simulink model "StateSpaceExe"  (R2018b)
settings: Solver=VariableStepAuto  StartTime=0.0  StopTime=100  RelTol=1e-3
values from neighbouring files (symbols this model uses):
  A = [-7.6258  0; 1  0]    [stateSpace.mat]    (also in stateSpaceData.mat; stateSpaceDataAntiWindup.mat)
  B = [1 0]    [stateSpace.mat]    (also in stateSpaceData.mat; stateSpaceDataAntiWindup.mat)
  C = [0 162.7435]    [stateSpace.mat]    (also in stateSpaceData.mat; stateSpaceDataAntiWindup.mat)
  D = 0    [stateSpace.mat]    (also in stateSpaceData.mat; stateSpaceDataAntiWindup.mat)
  K = [-3.4258 5.6 -0.014747132758]    [stateSpace.mat]    (also in stateSpaceData.mat = [-3.4258 5.6]; stateSpaceDataAntiWindup.mat = [82.3742 2600]; toStateSpace.m = [Kx(1) Kx(2)])
  Ki = -0.014747132758    [stateSpaceData.mat]    (also in stateSpaceDataAntiWindup.mat = 147.47132758; toStateSpace.m = Kx(3))
  L = [3.35099850771 0.334109810837]    [stateSpace.mat]    (also in stateSpaceData.mat = [0.0638134588478 0.0883242648708]; stateSpaceDataAntiWindup.mat = [191.93766157 2.22665851478]; toStateSpace.m = acker(A', C', [polo1, polo2])')
settings Model: Creator=lucas  LastModifiedBy=lucas

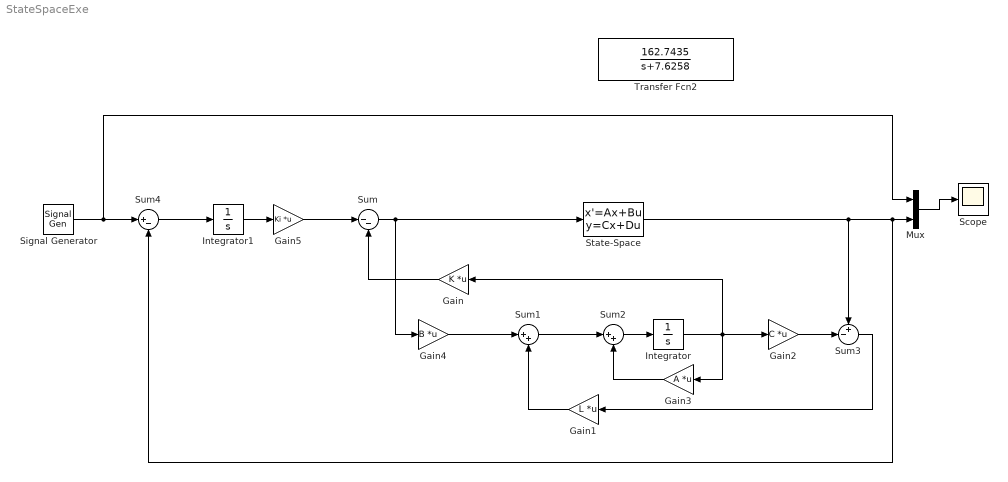
== system StateSpaceExe ==
  Gain : Gain  Gain=K  Multiplication=Matrix(K*u)
  Gain1 : Gain  Gain=L  Multiplication=Matrix(K*u)
  Gain2 : Gain  Gain=C  Multiplication=Matrix(K*u)
  Gain3 : Gain  Gain=A  Multiplication=Matrix(K*u)
  Gain4 : Gain  Gain=B  Multiplication=Matrix(K*u)
  Gain5 : Gain  Gain=Ki  Multiplication=Matrix(K*u)
  Integrator : Integrator
  Integrator1 : Integrator
  Mux : Mux  Inputs=2
  Scope : Scope
  Signal Generator : SignalGenerator  WaveForm=square  Amplitude=20  Frequency=0.1  Units=rad/sec
  State-Space : StateSpace  A=A  B=B  C=C  D=D  InitialCondition=0
  Sum : Sum  Inputs=|--
  Sum1 : Sum  Inputs=|++
  Sum2 : Sum  Inputs=|++
  Sum3 : Sum  Inputs=+-|
  Sum4 : Sum  Inputs=|+-
  Transfer Fcn2 : TransferFcn  Numerator=[162.7435]  Denominator="[1  7.6258]"
  wires:
  Mux/1 -> Scope/1
  Sum4/1 -> Integrator1/1
  Sum/1 -> State-Space/1, Gain4/1
  Gain2/1 -> Sum3/2
  Gain3/1 -> Sum2/2
  Sum2/1 -> Integrator/1
  Sum3/1 -> Gain1/1
  Gain1/1 -> Sum1/2
  Sum1/1 -> Sum2/1
  Gain4/1 -> Sum1/1
  Integrator/1 -> Gain/1, Gain3/1, Gain2/1
  Gain/1 -> Sum/2
  Signal Generator/1 -> Mux/1, Sum4/1
  State-Space/1 -> Sum3/1, Sum4/2, Mux/2
  Integrator1/1 -> Gain5/1
  Gain5/1 -> Sum/1
